simulink model "InnerLoop_Control"  (R2024b)
settings: configuration reference "csSingleInstance" (kept outside this file)
undefined symbols (not defined in the file): fbLoopGain
libraries: FilterLib x3, simulink x1
Description:
  | This model implements the multi-variable inner loop control (for pitch, roll, and yaw rate) of the helicopter flight control software.
settings Model: DataDictionary=DD_InnerLoop_Control.sldd  EnableAccessToBaseWorkspace=off  Creator=The MathWorks, Inc.  LastModifiedBy=The MathWorks, Inc.
settings ConfigSetRef: SourceName=csSingleInstance

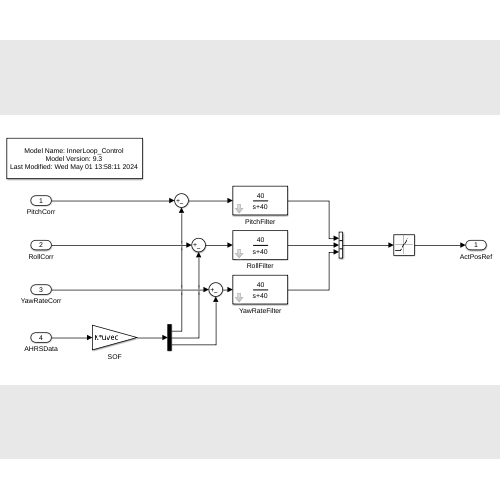
[thumbnail: Simulink's stored preview of the top-level diagram]
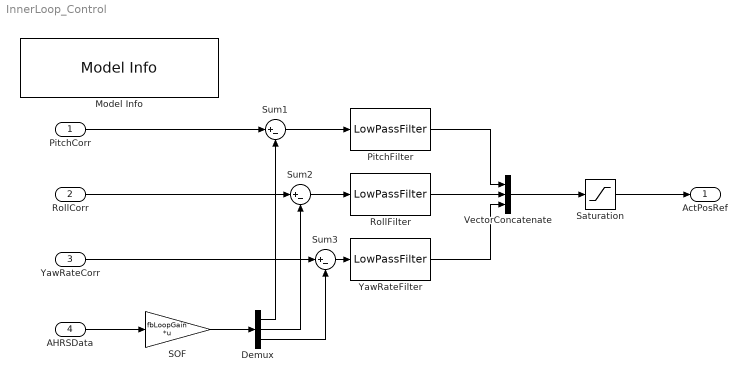
== system InnerLoop_Control ==
  PitchCorr : Inport  OutMin=-30  OutMax=30  OutDataTypeStr=double  PortDimensions=1  SampleTime=0.01
  RollCorr : Inport  Port=2  OutMin=-30  OutMax=30  OutDataTypeStr=double  PortDimensions=1  SampleTime=0.01
  YawRateCorr : Inport  Port=3  OutMin=-15  OutMax=15  OutDataTypeStr=double  PortDimensions=1  SampleTime=0.01
  AHRSData : Inport  Port=4  OutMin=-180  OutMax=180  OutDataTypeStr=double  PortDimensions=5  SampleTime=0.01
  Demux : Demux  Outputs=3
  Model Info : simulink/Model-Wide Utilities/Model Info  Frame=on  DisplayStringWithTags=|  HorizontalTextAlignment=Center  LeftAlignmentValue=0.5
      | Model Name: %<ModelName>
      | Model Version: %<ModelVersion>
      | Last Modified: %<LastModificationDate>
  PitchFilter : FilterLib/LowPassFilter  fq=40  ts=0.01
  RollFilter : FilterLib/LowPassFilter  fq=40  ts=0.01
  SOF : Gain  Gain=fbLoopGain  Multiplication=Matrix(K*u) (u vector)
  Saturation : Saturate  UpperLimit=0.1  LowerLimit=-0.1
  Sum1 : Sum  Inputs=|+-
  Sum2 : Sum  Inputs=|+-
  Sum3 : Sum  Inputs=|+-
  VectorConcatenate : Concatenate  NumInputs=3
  YawRateFilter : FilterLib/LowPassFilter  fq=40  ts=0.01
  ActPosRef : Outport  OutDataTypeStr=double  VectorParamsAs1DForOutWhenUnconnected=off
  wires:
  Sum2/1 -> RollFilter/1
  RollFilter/1 -> VectorConcatenate/2
  PitchCorr/1 -> Sum1/1
  Sum1/1 -> PitchFilter/1
  SOF/1 -> Demux/1
  RollCorr/1 -> Sum2/1
  YawRateCorr/1 -> Sum3/1
  Sum3/1 -> YawRateFilter/1
  Demux/1 -> Sum1/2
  Demux/2 -> Sum2/2
  Demux/3 -> Sum3/2
  AHRSData/1 -> SOF/1
  VectorConcatenate/1 -> Saturation/1
  YawRateFilter/1 -> VectorConcatenate/3
  PitchFilter/1 -> VectorConcatenate/1
  Saturation/1 -> ActPosRef/1
